simulink model "v2x_template"  (R2021b)
settings: Solver=FixedStepDiscrete  StartTime=0.0  StopTime=1000  RelTol=1e-3
libraries: commdigbbndpm3 x3, commsink2 x1, commrandsrc3 x1, commchan3 x1, dspstat3 x1, commseqgen3 x1
settings Model: DataTypeOverride=Off  Creator=jacob  LastModifiedBy=jacob
settings SolverCC: AlgebraicLoopSolver=TrustRegion
settings DataIOCC: LimitDataPoints=on  SaveOutput=off  SaveTime=off
settings OptimizationCC: BlockReduction=off  ConditionallyExecuteInputs=off  DefaultParameterBehavior=Inlined  LifeSpan=inf
settings DebuggingCC: AlgebraicLoopMsg=error  SingleTaskRateTransMsg=error  AllowSymbolicDim=off  StrictBusMsg=ErrorOnBusTreatedAsVector  SFUnexpectedBacktrackingDiag=warning  SFNoUnconditionalDefaultTransitionDiag=warning  SFExecutionAtInitializationDiag=none  SFMachineParentedDataDiag=warning  ArithmeticOperatorsInVariantConditions=warning
settings HardwareCC: ProdBitPerPointer=32  ProdBitPerSizeT=32  ProdBitPerPtrDiffT=32  ProdLargestAtomicFloat=None  ProdIntDivRoundTo=Undefined  ProdEndianess=Unspecified  ProdWordSize=32  ProdHWDeviceType=ASIC/FPGA->ASIC/FPGA  ProdEqTarget=off
settings SFSimCC: SimUseLocalCustomCode=off  CustomCodeUndefinedFunction=UseInterfaceOnly
settings RTWCC: RTWUseLocalCustomCode=off
settings CodeAppCC: StateflowObjectComments=on
settings GRTTargetCC: TargetLangStandard=C89/C90 (ANSI)
settings ConfigComp: CovScope=ReferencedModels  CovMetricSettings=dw  CovSaveCumulativeToWorkspaceVar=on  CovSaveSingleToWorkspaceVar=on  CovExternalEMLEnable=off  CovSFcnEnable=off

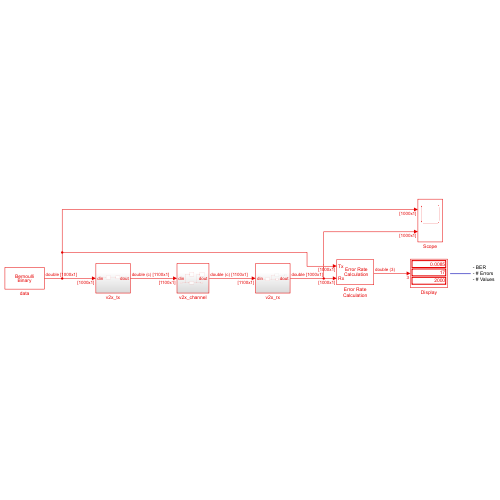
[thumbnail: Simulink's stored preview of the top-level diagram]
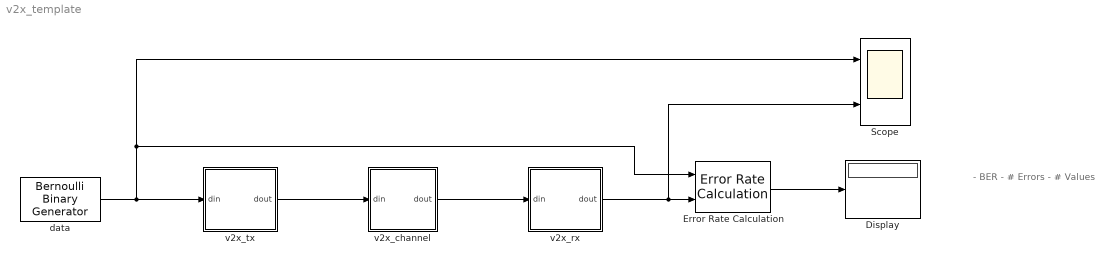
== system v2x_template ==
  note: - BER
      | - # Errors
      | - # Values
  Display : Display
  Error Rate Calculation : commsink2/Error Rate Calculation  N=0  st_delay=0  cp_mode=Entire frame  subframe=[]  PMode=Port  WsName=ErrorVec  RsMode2=off  stop=off  numErr=100  maxBits=1e6
  Scope : Scope  NumInputPorts=2
  data : commrandsrc3/Bernoulli Binary Generator  ProbabilityOfZero=0.5  SeedSource=Auto  Seed=0  SampleTime=1  SamplesPerFrame=1000  OutputDataType=double  SimulateUsing=Interpreted execution
  v2x_channel : Subsystem
  v2x_rx : Subsystem
  v2x_tx : Subsystem
  wires:
  data/1 -> Error Rate Calculation/1, Scope/1, v2x_tx/1(din)
  v2x_channel/1(dout) -> v2x_rx/1(din)
  v2x_tx/1(dout) -> v2x_channel/1(din)
  v2x_rx/1(dout) -> Error Rate Calculation/2, Scope/2
  Error Rate Calculation/1 -> Display/1

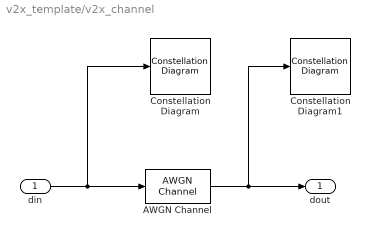
== system v2x_template/v2x_channel ==
  din : Inport
  AWGN Channel : commchan3/AWGN Channel  InputProcessing=Columns as channels (frame based)  seed=67  noiseMode="Signal to noise ratio  (Eb/No)"  EbNodB=5  EsNodB=10  SNRdB=10  bitsPerSym=1  Ps=1  Tsym=1  variance=1
  Constellation Diagram : ConstellationDiagram
  Constellation Diagram1 : ConstellationDiagram
  dout : Outport
  wires:
  AWGN Channel/1 -> Constellation Diagram1/1, dout/1
  din/1 -> Constellation Diagram/1, AWGN Channel/1

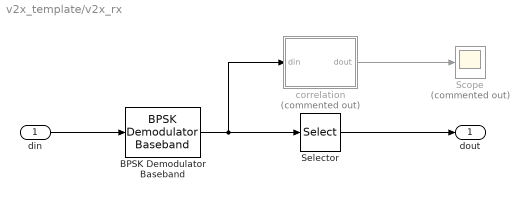
== system v2x_template/v2x_rx ==
  din : Inport
  BPSK Demodulator Baseband : commdigbbndpm3/BPSK Demodulator Baseband  DecType=Hard decision  VarSource=Dialog  Variance=1  Ph=pi  outDtype=Inherit via internal rule  derotateFactorWordLen=16  derotateFactorDataTypeStr=Inherit: Same word length as input  derotateFactorLastDataTypeStr=Inherit: Same word length as input
  Scope : Scope  Commented=on
  Selector : Selector  NumberOfDimensions=2  InputPortWidth=1  IndexOptions=Starting index (dialog),Starting index (dialog)  Indices=101,1  OutputSizes=1000,1
  correlation : Subsystem  Commented=on
  dout : Outport
  wires:
  BPSK Demodulator Baseband/1 -> correlation/1(din), Selector/1
  din/1 -> BPSK Demodulator Baseband/1
  Selector/1 -> dout/1
  correlation/1(dout) -> Scope/1

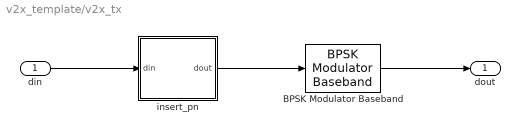
== system v2x_template/v2x_tx ==
  din : Inport
  BPSK Modulator Baseband : commdigbbndpm3/BPSK Modulator Baseband  Ph=pi  outDtype=double  outWordLen=16  outUDDataType=sfix(16)  outFracLenMode=Best precision  outFracLen=15  outDataTypeStr=double  outLastDataTypeStr=double
  insert_pn : Subsystem
  dout : Outport
  wires:
  insert_pn/1(dout) -> BPSK Modulator Baseband/1
  din/1 -> insert_pn/1(din)
  BPSK Modulator Baseband/1 -> dout/1

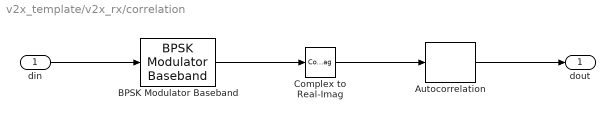
== system v2x_template/v2x_rx/correlation ==
  din : Inport
  Autocorrelation : dspstat3/Autocorrelation  AllPositiveLags=on  maxlag=1  bias=None  domain=Time  roundingMode=Floor  overflowMode=off  outputDataTypeStr=Inherit: Same as accumulator  outputMin=[]  outputMax=[]  outputLastDataTypeStr=Inherit: Same as accumulator
      settings: SourceProductBaseCode=DS
  BPSK Modulator Baseband : commdigbbndpm3/BPSK Modulator Baseband  Ph=pi  outDtype=double  outWordLen=16  outUDDataType=sfix(16)  outFracLenMode=Best precision  outFracLen=15  outDataTypeStr=double  outLastDataTypeStr=double
  Complex to Real-Imag : ComplexToRealImag  Output=Real
  dout : Outport
  wires:
  din/1 -> BPSK Modulator Baseband/1
  BPSK Modulator Baseband/1 -> Complex to Real-Imag/1
  Complex to Real-Imag/1 -> Autocorrelation/1
  Autocorrelation/1 -> dout/1

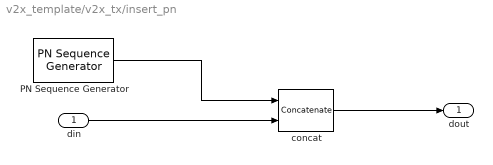
== system v2x_template/v2x_tx/insert_pn ==
  din : Inport
  PN Sequence Generator : commseqgen3/PN Sequence Generator  poly='z^6 + z + 1'  ini_sta=[0 0 0 0 0 1]  outBitMaskSource=Dialog parameter  shift=0  outVarSiz=off  maxOutSizeMode=Dialog parameter  maxOutSize=[10 1]  Ts=-1  sampPerFrame=100  reset=off  bitPackedOutputs=off  outDataType=double  numPackedBits=8  bitPackDataSigned=off  bitPackedOutDType=double
  concat : Concatenate  ConcatenateDimension=2
  dout : Outport
  wires:
  PN Sequence Generator/1 -> concat/1
  concat/1 -> dout/1
  din/1 -> concat/2
